simulink model "sla_pidctrl"  (R2015b)
settings: Solver=ode45  SolverMode=SingleTasking  StartTime=0.0  StopTime=10  RelTol=1e-3
libraries: simulink x1
settings Model: MinMaxOverflowLogging=MinMaxAndOverflow  Creator=at-mt  LastModifiedBy=amatsumo
settings DataIOCC: SaveFormat=Array  SignalLoggingSaveFormat=ModelDataLogs  SaveOutput=off  SignalLogging=off  SaveTime=off
settings OptimizationCC: BlockReduction=off  ConditionallyExecuteInputs=off  DefaultParameterBehavior=Inlined  ExpressionDepthLimit=2147483647
settings DebuggingCC: AlgebraicLoopMsg=error  UnderspecifiedInitializationDetection=Classic  MergeDetectMultiDrivingBlocksExec=none  SolverPrmCheckMsg=warning  MultiTaskRateTransMsg=warning  SingleTaskRateTransMsg=warning  FcnCallInpInsideContextMsg=UseLocalSettings  StateNameClashWarn=warning
settings HardwareCC: ProdBitPerPointer=32  ProdLargestAtomicFloat=None  ProdIntDivRoundTo=Undefined  ProdEndianess=Unspecified  ProdWordSize=32  ProdHWDeviceType=ASIC/FPGA->ASIC/FPGA  ProdEqTarget=off
settings GRTTargetCC: GeneratePreprocessorConditionals=Disable all  CombineOutputUpdateFcns=off  GRTInterface=on
settings ConfigComp: CovModelRefEnable=Off  CovSFcnEnable=off

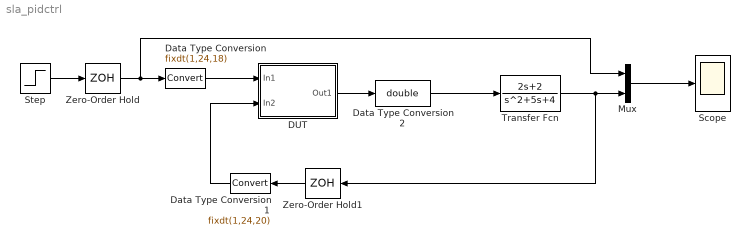
== system sla_pidctrl ==
  DUT : Subsystem
  Data Type Conversion : DataTypeConversion  OutDataTypeStr=fixdt(1,24,18)  RndMeth=Nearest
  Data Type Conversion1 : DataTypeConversion  OutDataTypeStr=fixdt(1,24,20)  RndMeth=Nearest
  Data Type Conversion2 : DataTypeConversion  OutDataTypeStr=double  RndMeth=Nearest
  Mux : Mux  Inputs=2
  Scope : Scope
  Step : Step  SampleTime=0
  Transfer Fcn : TransferFcn  Numerator=[2 2]  Denominator=[1 5 4]
  Zero-Order Hold : ZeroOrderHold  SampleTime=1/1000
  Zero-Order Hold1 : ZeroOrderHold  SampleTime=1/1000
  wires:
  Step/1 -> Zero-Order Hold/1
  DUT/1(Out1) -> Data Type Conversion2/1
  Zero-Order Hold/1 -> Mux/1, Data Type Conversion/1
  Transfer Fcn/1 -> Mux/2, Zero-Order Hold1/1
  Mux/1 -> Scope/1
  Zero-Order Hold1/1 -> Data Type Conversion1/1
  Data Type Conversion/1 -> DUT/1(In1)
  Data Type Conversion1/1 -> DUT/2(In2)
  Data Type Conversion2/1 -> Transfer Fcn/1

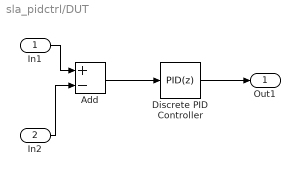
== system sla_pidctrl/DUT ==
  In1 : Inport
  In2 : Inport  Port=2
  Add : Sum  Inputs=+-  OutDataTypeStr=fixdt(1,24,18)  RndMeth=Nearest
  Discrete PID Controller : simulink/Continuous/PID Controller  Controller=PID  TimeDomain=Discrete-time  SampleTime=1/1000  IntegratorMethod=Forward Euler  FilterMethod=Forward Euler  Form=Parallel  UseFilter=on  ControllerParametersSource=internal  P=1.25134279272754  I=10.6219913651335  D=-0.130168547266747  N=9.52685147948318  InitialConditionSource=internal  InitialConditionForIntegrator=0  InitialConditionForFilter=0  ExternalReset=none  LimitOutput=on  UpperSaturationLimit=32  LowerSaturationLimit=-32  LinearizeAsGain=off  AntiWindupMode=none  Kb=1  TrackingMode=off  Kt=1  RndMeth=Nearest  SaturateOnIntegerOverflow=on  PParamMin=0  PParamMax=1.9  PParamDataTypeStr=fixdt(0,6,5)  IParamMin=0  IParamMax=20  IParamDataTypeStr=fixdt(0,10,5)  DParamMin=-1.9  DParamMax=1.9  DParamDataTypeStr=fixdt(1,6,4)  NParamMin=0  NParamMax=10  NParamDataTypeStr=fixdt(0,5,1)  KbParamMin=[]  KbParamMax=[]  KtParamMin=[]  KtParamMax=[]  POutMin=-1  POutMax=1.9  POutDataTypeStr=fixdt(1,24,22)  PGainOutDataTypeStr=fixdt(1,24,22)  PProdOutDataTypeStr=fixdt(1,24,22)  IOutMin=-10  IOutMax=7  IOutDataTypeStr=fixdt(1,24,18)  IGainOutDataTypeStr=fixdt(1,24,18)  IProdOutDataTypeStr=fixdt(1,24,18)  DOutMin=-1.9  DOutMax=1.9  DOutDataTypeStr=fixdt(1,24,22)  DGainOutDataTypeStr=fixdt(1,24,22)  DProdOutDataTypeStr=fixdt(1,24,22)  NOutMin=0  NOutMax=10  NOutDataTypeStr=fixdt(1,24,19)  NGainOutDataTypeStr=fixdt(1,24,19)  NProdOutDataTypeStr=fixdt(1,24,19)  KbOutMin=[]  KbOutMax=[]  KtOutMin=[]  KtOutMax=[]  IntegratorOutMin=0  IntegratorOutMax=2  IntegratorOutDataTypeStr=fixdt(1,24,21)  FilterOutMin=-1  FilterOutMax=0.9  FilterOutDataTypeStr=fixdt(1,24,23)  SumOutMin=-10  SumOutMax=16  SumOutDataTypeStr=fixdt(1,24,18)  SumI1OutMin=[]  SumI1OutMax=[]  SumI2OutMin=[]  SumI2OutMax=[]  SumI3OutMin=[]  SumI3OutMax=[]  SumDOutMin=-1  SumDOutMax=1.9  SumDOutDataTypeStr=fixdt(1,24,22)  SaturationOutMin=[]  SaturationOutMax=[]  IntegratorContinuousStateAttributes=''  IntegratorStateMustResolveToSignalObject=off  IntegratorRTWStateStorageClass=Auto  FilterContinuousStateAttributes=''  FilterStateMustResolveToSignalObject=off  FilterRTWStateStorageClass=Auto  DifferentiatorICPrevScaledInput=0  DifferentiatorOutMin=[]  DifferentiatorOutMax=[]
  Out1 : Outport
  wires:
  Add/1 -> Discrete PID Controller/1
  In1/1 -> Add/1
  Discrete PID Controller/1 -> Out1/1
  In2/1 -> Add/2
